simulink model "VTOL_sim"  (R2015a)
settings: Solver=ode45  StartTime=0.0  StopTime=200  RelTol=1e-3
InitFcn:
  | param
undefined symbols (not defined in the file or in its folder): drawVTOL, P
settings Model: Creator=beard  LastModifiedBy=wynn4
settings DataIOCC: SignalLoggingSaveFormat=ModelDataLogs
settings OptimizationCC: ExpressionDepthLimit=2147483647  InitFltsAndDblsToZero=on
settings DebuggingCC: UnderspecifiedInitializationDetection=Classic  MergeDetectMultiDrivingBlocksExec=none  SolverPrmCheckMsg=warning  FcnCallInpInsideContextMsg=UseLocalSettings  StateNameClashWarn=warning
settings GRTTargetCC: CombineOutputUpdateFcns=off  GRTInterface=on

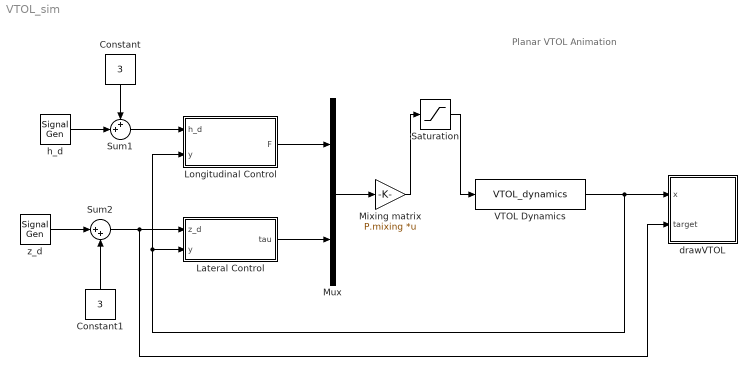
== system VTOL_sim ==
  note: Planar VTOL Animation
  Constant : Constant  Value=3
  Constant1 : Constant  Value=3
  Lateral Control : Subsystem
  Longitudinal Control : Subsystem
  Mixing matrix : Gain  Gain=P.mixing  Multiplication=Matrix(K*u)
  Mux : Mux  Inputs=2
  Saturation : Saturate  UpperLimit=10  LowerLimit=0
  Sum1 : Sum  Inputs=++|
  Sum2 : Sum  Inputs=|++
  VTOL Dynamics : S-Function  FunctionName=VTOL_dynamics  Parameters=AP
  drawVTOL : Subsystem
      mask Display: image(imread('tv.jpg'))
  h_d : SignalGenerator  WaveForm=square  Amplitude=2.5  Frequency=.02
  z_d : SignalGenerator  WaveForm=square  Amplitude=2.5  Frequency=.008
  wires:
  VTOL Dynamics/1 -> Longitudinal Control/2(y), Lateral Control/2(y), drawVTOL/1(x)
  Mux/1 -> Mixing matrix/1
  Longitudinal Control/1(F) -> Mux/1
  Lateral Control/1(tau) -> Mux/2
  Constant/1 -> Sum1/1
  Sum1/1 -> Longitudinal Control/1(h_d)
  h_d/1 -> Sum1/2
  Sum2/1 -> drawVTOL/2(target), Lateral Control/1(z_d)
  z_d/1 -> Sum2/1
  Constant1/1 -> Sum2/2
  Mixing matrix/1 -> Saturation/1
  Saturation/1 -> VTOL Dynamics/1

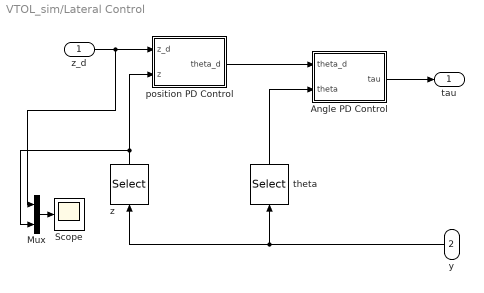
== system VTOL_sim/Lateral Control ==
  z_d : Inport
  y : Inport  Port=2
  "Angle PD Control " : Subsystem
  Mux : Mux  Inputs=2
  Scope : Scope
      settings: YMin=-1  YMax=7  SaveName=ScopeData2
  position PD Control : Subsystem
  theta : Selector  InputPortWidth=3  Indices=[3]
  z : Selector  InputPortWidth=3  Indices=[1]
  tau : Outport
  wires:
  y/1 -> z/1, theta/1
  position PD Control/1(theta_d) -> "Angle PD Control "/1(theta_d)
  theta/1 -> "Angle PD Control "/2(theta)
  z_d/1 -> Mux/1, position PD Control/1(z_d)
  z/1 -> Mux/2, position PD Control/2(z)
  "Angle PD Control "/1(tau) -> tau/1
  Mux/1 -> Scope/1

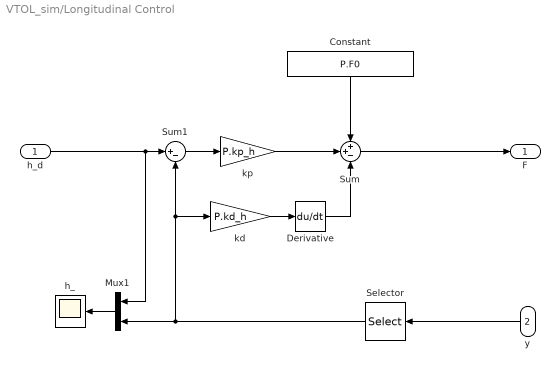
== system VTOL_sim/Longitudinal Control ==
  h_d : Inport
  y : Inport  Port=2
  Constant : Constant  Value=P.F0
  Derivative : Derivative
  Mux1 : Mux  Inputs=2
  Selector : Selector  InputPortWidth=3  Indices=[2]
  Sum : Sum  Inputs=++-
  Sum1 : Sum  Inputs=|+-
  h_ : Scope
      settings: TimeRange=200  YMin=0  YMax=6
  kd : Gain  Gain=P.kd_h
  kp : Gain  Gain=P.kp_h
  F : Outport
  wires:
  Selector/1 -> kd/1, Sum1/2, Mux1/2
  Derivative/1 -> Sum/3
  Sum/1 -> F/1
  Mux1/1 -> h_/1
  kd/1 -> Derivative/1
  Constant/1 -> Sum/1
  h_d/1 -> Sum1/1, Mux1/1
  Sum1/1 -> kp/1
  y/1 -> Selector/1
  kp/1 -> Sum/2

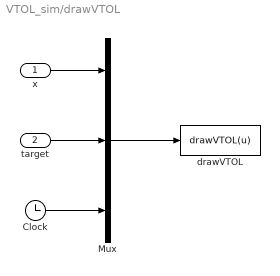
== system VTOL_sim/drawVTOL ==
  x : Inport
  target : Inport  Port=2
  Clock : Clock
  Mux : Mux  Inputs=3
  drawVTOL : MATLABFcn  MATLABFcn=drawVTOL(u)  OutputDimensions=0  SampleTime=0.1
  wires:
  Mux/1 -> drawVTOL/1
  x/1 -> Mux/1
  Clock/1 -> Mux/3
  target/1 -> Mux/2

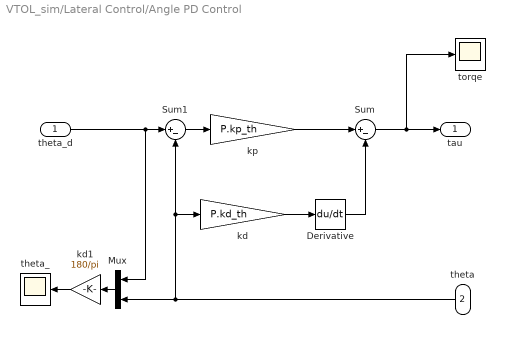
== system VTOL_sim/Lateral Control/Angle PD Control  ==
  theta_d : Inport
  theta : Inport  Port=2
  Derivative : Derivative
  Mux : Mux  Inputs=2
  Sum : Sum  Inputs=|+-
  Sum1 : Sum  Inputs=|+-
  kd : Gain  Gain=P.kd_th
  kd1 : Gain  Gain=180/pi
  kp : Gain  Gain=P.kp_th
  theta_ : Scope
      settings: TimeRange=200  YMin=-1.5  YMax=1.5
  torqe : Scope
      settings: YMin=0.15  YMax=1
  tau : Outport
  wires:
  theta_d/1 -> Sum1/1, Mux/1
  Sum/1 -> torqe/1, tau/1
  theta/1 -> kd/1, Sum1/2, Mux/2
  Sum1/1 -> kp/1
  kd1/1 -> theta_/1
  kp/1 -> Sum/1
  Mux/1 -> kd1/1
  kd/1 -> Derivative/1
  Derivative/1 -> Sum/2

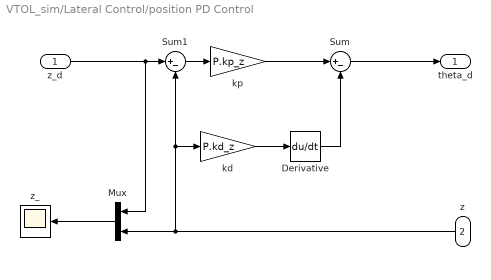
== system VTOL_sim/Lateral Control/position PD Control ==
  z_d : Inport
  z : Inport  Port=2
  Derivative : Derivative
  Mux : Mux  Inputs=2
  Sum : Sum  Inputs=|+-
  Sum1 : Sum  Inputs=|+-
  kd : Gain  Gain=P.kd_z
  kp : Gain  Gain=P.kp_z
  z_ : Scope
      settings: TimeRange=200  YMin=-1  YMax=7
  theta_d : Outport
  wires:
  z_d/1 -> Sum1/1, Mux/1
  Sum/1 -> theta_d/1
  z/1 -> kd/1, Sum1/2, Mux/2
  Sum1/1 -> kp/1
  Mux/1 -> z_/1
  kp/1 -> Sum/1
  kd/1 -> Derivative/1
  Derivative/1 -> Sum/2
